simulink model "Sudarshan_1_lab_7"  (R2022b)
settings: Solver=VariableStepAuto  StartTime=0.0  StopTime=1  RelTol=1e-3
settings Model: Creator=year2  LastModifiedBy=year2

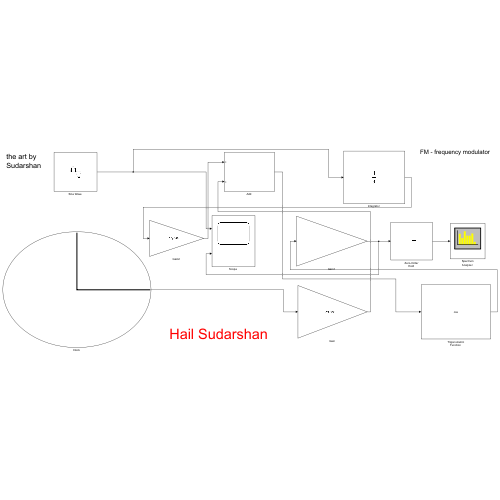
[thumbnail: Simulink's stored preview of the top-level diagram]
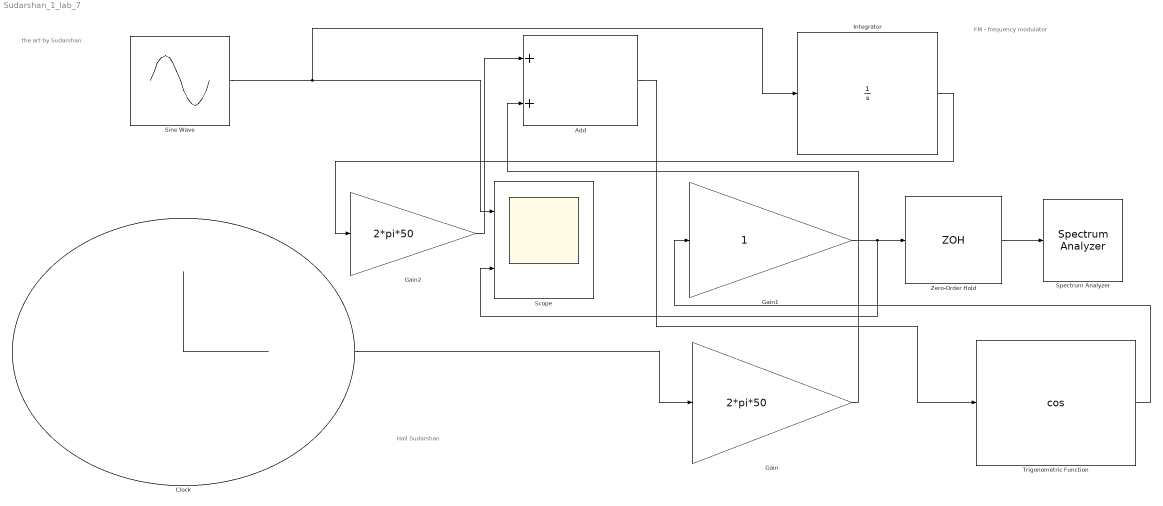
== system Sudarshan_1_lab_7 ==
  note: Hail Sudarshan
  note: FM - frequency modulator
  note: the art by Sudarshan
  "Add " : Sum
  "Clock " : Clock
  "Gain " : Gain  Gain=2*pi*50
  "Gain1 " : Gain
  "Gain2 " : Gain  Gain=2*pi*50
  "Integrator " : Integrator
  "Scope " : Scope  NumInputPorts=2
  "Sine Wave " : Sin  Frequency=10  SampleTime=0.0000001  VectorParams1D=off
  "Spectrum Analyzer " : SpectrumAnalyzer
  "Trigonometric Function " : Trigonometry  Operator=cos
  "Zero-Order Hold " : ZeroOrderHold  SampleTime=-1
  wires:
  "Sine Wave "/1 -> "Integrator "/1, "Scope "/1
  "Clock "/1 -> "Gain "/1
  "Gain1 "/1 -> "Scope "/2, "Zero-Order Hold "/1
  "Zero-Order Hold "/1 -> "Spectrum Analyzer "/1
  "Gain "/1 -> "Add "/2
  "Gain2 "/1 -> "Add "/1
  "Integrator "/1 -> "Gain2 "/1
  "Add "/1 -> "Trigonometric Function "/1
  "Trigonometric Function "/1 -> "Gain1 "/1
